simulink model "satellite_GVE_per_model_withMPC_sim"  (R2021a)
settings: Solver=VariableStepAuto  StartTime=0  StopTime=43200  FixedStep=1  RelTol=1e-3
values from neighbouring files (symbols this model uses):
  a = a_ini    (= 7367700)    [Satellite_MPC2.m]
  a_ini = (960e3+1019e3)/2+R_e    (= 7367700)    [Satellite_MPC2.m]
  Cd = 2.2    [Satellite_MPC2.m]
  e = e_ini    (= 0.0039866)    [Satellite_MPC2.m]
  e_ini = 0.0039866    [Satellite_MPC2.m]
  i = i_ini    [Satellite_MPC2.m]
  i_ini = 82.9236/180*pi()    [Satellite_MPC2.m]
  J2 = 1082.63e-6    (= 0.00108263)    [Satellite_MPC2.m]
  K = 2    [Satellite_MPC2.m]
  m_s = 27    [Satellite_MPC2.m]
  meu = G*m_e    (= 397865500000000)    [Satellite_MPC2.m]
  Ohm = Ohm_ini    [Satellite_MPC2.m]
  Ohm_ini = 272.9481/180*pi()    [Satellite_MPC2.m]
  p_solar = 4.65e-06    [Satellite_MPC2.m]
  R_e = 6378.2e3    (= 6378200)    [Satellite_MPC2.m]
  s = 0.2*0.2    (= 0.04)    [Satellite_MPC2.m]
  theta = theta_ini    (= 0)    [Satellite_MPC2.m]
  w = w_ini    [Satellite_MPC2.m]
  w_ini = 297.2910/180*pi()    [Satellite_MPC2.m]
libraries: mpclib x1
settings Model: OrderedModelArguments=off  Creator=18214  LastModifiedBy=18214

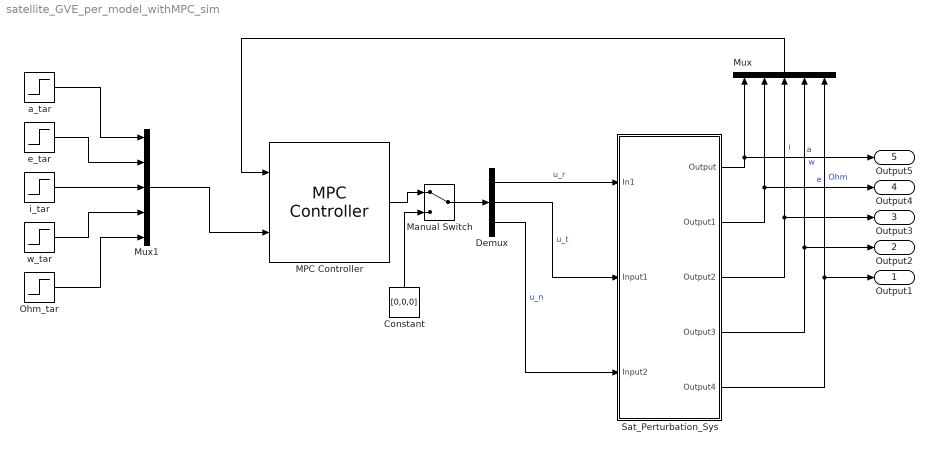
== system satellite_GVE_per_model_withMPC_sim ==
  Constant : Constant  Value=[0,0,0]
  Demux : Demux  Outputs=3
  MPC Controller : mpclib/MPC Controller  SCDEnableBlockLinearizationSpecification=on  mpcobj=mpc_per_exclude  is_multiple=0  enable_value=0  return_u0=off  updateMPCinCallerWorkspace=on  md_inport=off  mv_inport=off  uref_inport=off  return_cost=off  return_mvseq=off  return_qpstatus=off  return_xseq=off  return_state=off  return_ovseq=off  state_inport=off  umin_inport=off  umax_inport=off  ymin_inport=off  ymax_inport=off  cc_inport=off  ywt_inport=off  uwt_inport=off  duwt_inport=off  rhoeps_inport=off  pm_inport=off  MaximumP=10  HorizonChoice=FixedHorizon  n_ts=0.001  n_p=15  n_mv=3  n_md=0  n_ud=0  n_mo=5  n_uo=0  BlockDataType=double  SampleTimeInherited=off  switch_inport=off
  Manual Switch : ManualSwitch
  Mux : Mux  Inputs=5
  Mux1 : Mux  Inputs=5
  Ohm_tar : Step  Time=0  After=Ohm_ini  SampleTime=0
  Sat_Perturbation_Sys : Subsystem
  a_tar : Step  Time=0  After=a_ini  SampleTime=0
  e_tar : Step  Time=0  After=e_ini  SampleTime=0
  i_tar : Step  Time=0  After=i_ini  SampleTime=0
  w_tar : Step  Time=0  After=w_ini  SampleTime=0
  Output1 : Outport
  Output2 : Outport  Port=2
  Output3 : Outport  Port=3
  Output4 : Outport  Port=4
  Output5 : Outport  Port=5
  wires:
  Demux/2 -> Sat_Perturbation_Sys/2(Input1)  "u_t"
  Demux/3 -> Sat_Perturbation_Sys/3(Input2)  "u_n"
  Sat_Perturbation_Sys/1(Output) -> Mux/1, Output5/1  "a"
  Sat_Perturbation_Sys/2(Output1) -> Mux/2, Output4/1  "e"
  Sat_Perturbation_Sys/3(Output2) -> Mux/3, Output3/1  "i"
  Sat_Perturbation_Sys/4(Output3) -> Mux/4, Output2/1  "w"
  Demux/1 -> Sat_Perturbation_Sys/1(In1)  "u_r"
  Sat_Perturbation_Sys/5(Output4) -> Mux/5, Output1/1  "Ohm"
  MPC Controller/1 -> Manual Switch/1
  Mux/1 -> MPC Controller/1
  Mux1/1 -> MPC Controller/2
  a_tar/1 -> Mux1/1
  e_tar/1 -> Mux1/2
  i_tar/1 -> Mux1/3
  w_tar/1 -> Mux1/4
  Ohm_tar/1 -> Mux1/5
  Manual Switch/1 -> Demux/1
  Constant/1 -> Manual Switch/2

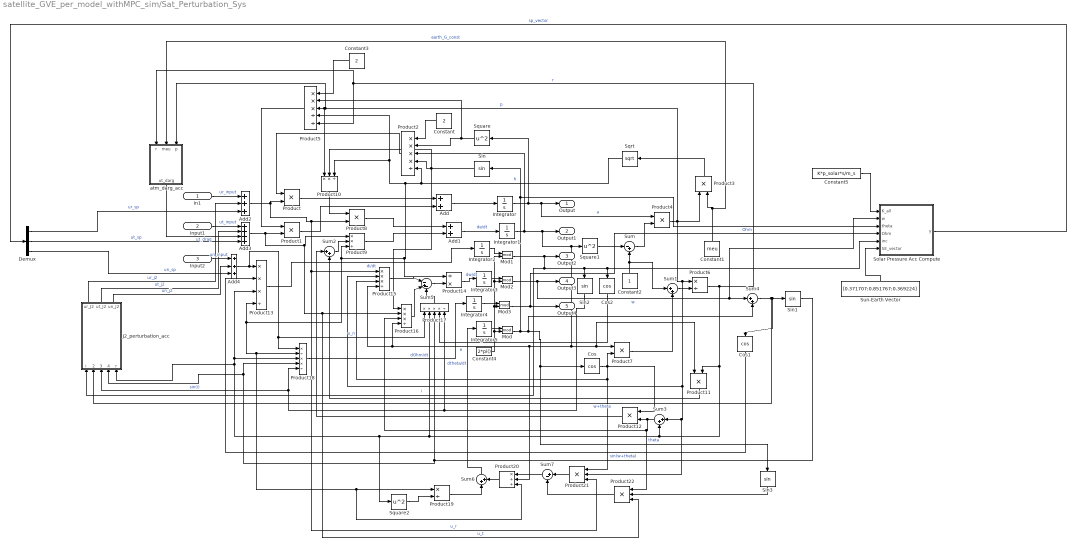
== system satellite_GVE_per_model_withMPC_sim/Sat_Perturbation_Sys ==
  In1 : Inport
  Input1 : Inport  Port=2
  Input2 : Inport  Port=3
  Add : Sum
  Add1 : Sum
  Add2 : Sum  Inputs=+++
  Add3 : Sum  Inputs=++++
  Add4 : Sum  Inputs=+++
  Constant : Constant  Value=2
  Constant1 : Constant  Value=meu
  Constant2 : Constant
  Constant3 : Constant  Value=2
  Constant4 : Constant  Value=2*pi()
  Constant5 : Constant  Value=K*p_solar*s/m_s
  Cos : Trigonometry  Operator=cos
  Cos1 : Trigonometry  Operator=cos
  Cos2 : Trigonometry  Operator=cos
  Demux : Demux  Outputs=3
  Integrator : Integrator  InitialCondition=a  LimitOutput=on  LowerSaturationLimit=R_e
  Integrator1 : Integrator  InitialCondition=e  LimitOutput=on  UpperSaturationLimit=1  LowerSaturationLimit=0
  Integrator2 : Integrator  InitialCondition=i  UpperSaturationLimit=312.5963  LowerSaturationLimit=-312.5963
  Integrator3 : Integrator  InitialCondition=w  UpperSaturationLimit=312.5963  LowerSaturationLimit=-312.5963
  Integrator4 : Integrator  InitialCondition=Ohm  UpperSaturationLimit=312.5963  LowerSaturationLimit=-312.5963
  Integrator5 : Integrator  InitialCondition=theta  UpperSaturationLimit=312.5963  LowerSaturationLimit=-312.5963
  J2_perturbation_acc : Subsystem
  Mod{,1..3} (4 alike) : Math  Operator=mod  SaturateOnIntegerOverflow=on
  Product{,1,3..4,7..8,11..12} (8 alike) : Product
  Product10 : Product  Inputs=**/
  Product13 : Product  Inputs=***/
  Product14 : Product  Inputs=/*
  Product15 : Product  Inputs=***/
  Product16 : Product  Inputs=***/
  Product17 : Product  Inputs=****/
  Product18 : Product  Inputs=*/**/
  Product19 : Product  Inputs=*/
  Product2 : Product  Inputs=****/
  Product20 : Product  Inputs=*//
  Product21 : Product  Inputs=***
  Product22 : Product  Inputs=***
  Product5 : Product  Inputs=***//
  Product6 : Product  Inputs=*/
  Product9 : Product  Inputs=**/
  Sin{,1..3} (4 alike) : Trigonometry
  Solar Pressure Acc Compute : MATLAB Function  TreatAsAtomicUnit=on
  Sqrt : Sqrt  SaturateOnIntegerOverflow=on
  Square : Math  Operator=square  SaturateOnIntegerOverflow=on
  Square1 : Math  Operator=square  SaturateOnIntegerOverflow=on
  Square2 : Math  Operator=square  SaturateOnIntegerOverflow=on
  Sum : Sum  Inputs=|-+
  Sum{1..4,6} (5 alike) : Sum  Inputs=|++
  Sum5 : Sum  Inputs=|-+-
  Sum7 : Sum  Inputs=|+-
  Sun-Earth Vector : Constant  Value=[0.371707;0.851767;0.369224]
  atm_darg_acc : Subsystem
  Output : Outport
  Output1 : Outport  Port=2
  Output2 : Outport  Port=3
  Output3 : Outport  Port=4
  Output4 : Outport  Port=5
  wires:
  Integrator/1 -> Output/1, Product4/1, Square/1  "a"
  Square2/1 -> Product19/2
  Product2/1 -> Product/1
  Mod/1 -> Sin/1, Solar Pressure Acc Compute/3(theta), Sin3/1, Cos/1, Sum4/2  "theta"
  Sin1/1 -> Product18/4, J2_perturbation_acc/4(sin(w+theta)), Product17/3  "sin(w+theta)"
  Product21/1 -> Sum7/1
  Sum5/1 -> Product14/2
  Cos/1 -> Product21/1, Product15/3, Product12/1, Product7/2
  Product4/1 -> Product15/2, Product21/2, Sum3/1, Product6/1, atm_darg_acc/3(p), Product10/1, Product5/3, Product3/1  "p"
  Cos2/1 -> Product17/4
  Sin/1 -> Product16/1, Product10/2, Product2/4
  Sqrt/1 -> Product10/3, Product5/4, Product14/1, Product13/4, Product20/3, Product19/1, Product18/2, Product9/3, Product2/5  "h"
  Product12/1 -> Sum2/1
  Sum/1 -> Product4/2
  Sum3/1 -> Product22/1, Product16/3, Product12/2
  Sum7/1 -> Product20/1
  Product1/1 -> Add/2
  Product22/1 -> Sum7/2
  Add2/1 -> Product/2, Product21/3, Product15/1, Product8/2  "u_r"
  Product7/1 -> Sum1/2
  Product5/1 -> Product1/1
  Sin3/1 -> Product22/2
  Product15/1 -> Sum5/1
  Integrator1/1 -> Product2/3, Output1/1, Square1/1, Product7/1, Product11/1, Product20/2, Product16/4, Product15/4  "e"
  Sum1/1 -> Product6/2
  Cos1/1 -> Product13/2
  Product19/1 -> Sum6/1
  Product8/1 -> Add1/1
  Product6/1 -> atm_darg_acc/1(r), Product5/5, Square2/1, J2_perturbation_acc/5(r), Product13/3, Product18/3, Product17/2, Sum3/2, Product11/2  "r"
  Constant2/1 -> Sum/2, Sum1/1
  Square/1 -> Product5/2, Product2/2
  Product11/1 -> Sum2/2
  Product/1 -> Add/1
  Mod1/1 -> Output2/1, Solar Pressure Acc Compute/5(inc), Cos2/1, Sin2/1, J2_perturbation_acc/1(i)  "i"
  Sin2/1 -> Product18/5, J2_perturbation_acc/3(sin(i)), Product17/5  "sin(i)"
  Product17/1 -> Sum5/3
  Product16/1 -> Sum5/2
  Sum6/1 -> Integrator5/1  "dtheta/dt"
  Product10/1 -> Product8/1
  Product9/1 -> Add1/2
  Sum4/1 -> Sin1/1, Cos1/1, J2_perturbation_acc/2(w+theta)  "w+theta"
  Product20/1 -> Sum6/2
  Mod2/1 -> Solar Pressure Acc Compute/2(w), Sum4/1, Output3/1  "w"
  Add3/1 -> Product22/3, Product16/2, Product9/1, Product1/2  "u_t"
  Constant/1 -> Product2/1
  Sum2/1 -> Product9/2
  Product14/1 -> Integrator3/1  "dw/dt"
  Square1/1 -> Sum/1
  Add4/1 -> Product18/1, Product17/1, Product13/1  "u_n"
  Product13/1 -> Integrator2/1  "di/dt"
  Constant1/1 -> atm_darg_acc/2(meu), Product3/2  "earth_G_const"
  Mod3/1 -> Solar Pressure Acc Compute/4(Ohm), Output4/1  "Ohm"
  Product18/1 -> Integrator4/1  "dOhm/dt"
  Add1/1 -> Integrator1/1  "de/dt"
  Constant3/1 -> Product5/1
  Product3/1 -> Sqrt/1
  Integrator5/1 -> Mod/1
  Constant4/1 -> Mod3/2, Mod2/2, Mod1/2, Mod/2
  In1/1 -> Add2/1  "ur_input"
  Input1/1 -> Add3/1  "ut_input"
  Input2/1 -> Add4/1  "un_input"
  atm_darg_acc/1(ut_darg) -> Add3/3  "ut_drag"
  J2_perturbation_acc/1(ur_J2) -> Add2/2  "ur_j2"
  J2_perturbation_acc/2(ut_J2) -> Add3/2  "ut_j2"
  J2_perturbation_acc/3(un_J2) -> Add4/2  "un_j2"
  Add/1 -> Integrator/1
  Integrator2/1 -> Mod1/1
  Integrator3/1 -> Mod2/1
  Integrator4/1 -> Mod3/1
  Sun-Earth Vector/1 -> Solar Pressure Acc Compute/6(SE_vector)
  Constant5/1 -> Solar Pressure Acc Compute/1(K_all)
  Solar Pressure Acc Compute/1(y) -> Demux/1  "sp_vector"
  Demux/1 -> Add2/3  "ur_sp"
  Demux/2 -> Add3/4  "ut_sp"
  Demux/3 -> Add4/3  "un_sp"

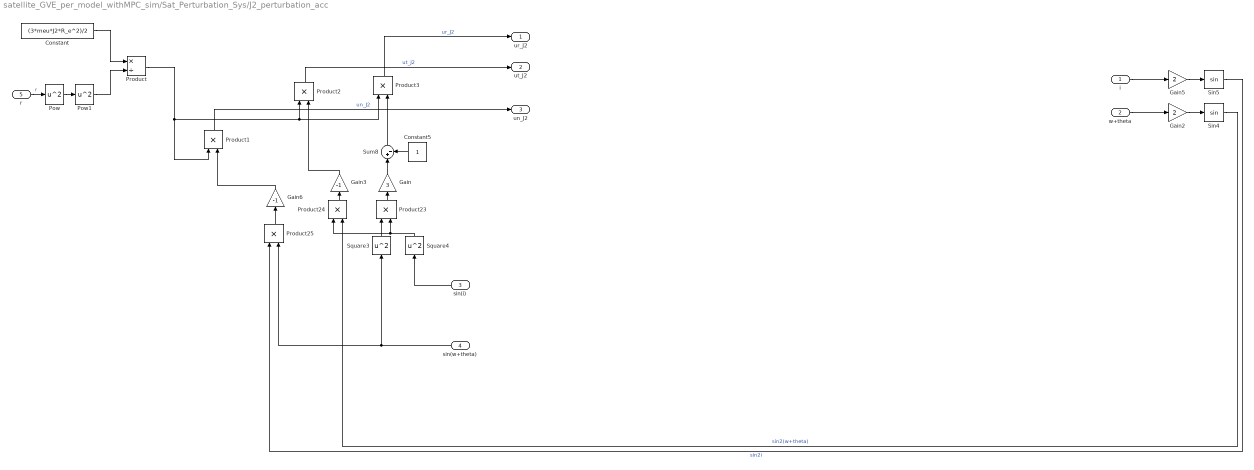
== system satellite_GVE_per_model_withMPC_sim/Sat_Perturbation_Sys/J2_perturbation_acc ==
  i : Inport
  w+theta : Inport  Port=2
  sin(i) : Inport  Port=3
  sin(w+theta) : Inport  Port=4
  r : Inport  Port=5
  Constant : Constant  Value=(3*meu*J2*R_e^2)/2
  Constant5 : Constant
  Gain : Gain  Gain=3
  Gain2 : Gain  Gain=2
  Gain3 : Gain  Gain=-1
  Gain5 : Gain  Gain=2
  Gain6 : Gain  Gain=-1
  Pow : Math  Operator=square  RndMeth=Zero  SaturateOnIntegerOverflow=on
  Pow1 : Math  Operator=square  RndMeth=Zero  SaturateOnIntegerOverflow=on
  Product : Product  Inputs=*/
  Product{1..3,23..25} (6 alike) : Product
  Sin4 : Trigonometry
  Sin5 : Trigonometry
  Square3 : Math  Operator=square  SaturateOnIntegerOverflow=on
  Square4 : Math  Operator=square  SaturateOnIntegerOverflow=on
  Sum8 : Sum  Inputs=|+-
  ur_J2 : Outport
  ut_J2 : Outport  Port=2
  un_J2 : Outport  Port=3
  wires:
  Gain6/1 -> Product1/2
  Square4/1 -> Product23/2, Product24/1
  i/1 -> Gain5/1
  Square3/1 -> Product23/1
  Sin4/1 -> Product24/2  "sin2(w+theta)"
  Sum8/1 -> Product3/2
  Product3/1 -> ur_J2/1  "ur_J2"
  Gain5/1 -> Sin5/1
  Gain3/1 -> Product2/2
  w+theta/1 -> Gain2/1
  Gain/1 -> Sum8/1
  Product23/1 -> Gain/1
  sin(w+theta)/1 -> Product25/2, Square3/1
  Constant5/1 -> Sum8/2
  Sin5/1 -> Product25/1  "sin2i"
  Gain2/1 -> Sin4/1
  Product25/1 -> Gain6/1
  Product24/1 -> Gain3/1
  Product2/1 -> ut_J2/1  "ut_J2"
  sin(i)/1 -> Square4/1
  Product1/1 -> un_J2/1  "un_J2"
  r/1 -> Pow/1  "r"
  Pow1/1 -> Product/2
  Constant/1 -> Product/1
  Product/1 -> Product3/1, Product2/1, Product1/1
  Pow/1 -> Pow1/1

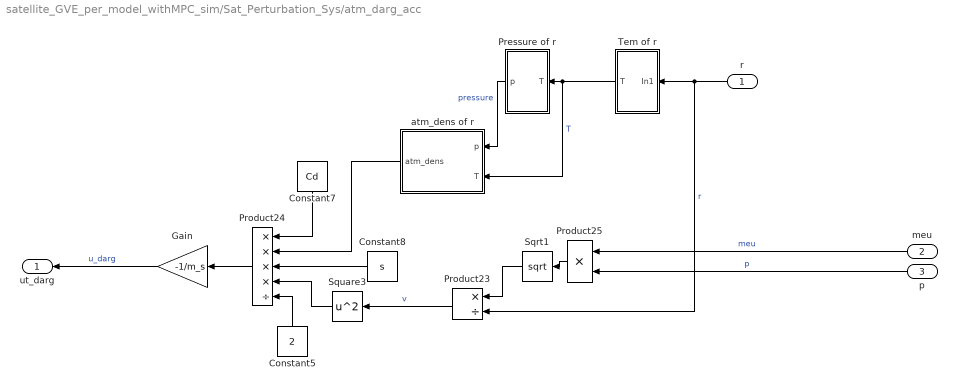
== system satellite_GVE_per_model_withMPC_sim/Sat_Perturbation_Sys/atm_darg_acc ==
  r : Inport
  meu : Inport  Port=2
  p : Inport  Port=3
  Constant5 : Constant  Value=2
  Constant7 : Constant  Value=Cd
  Constant8 : Constant  Value=s
  Gain : Gain  Gain=-1/m_s
  Pressure of r : Subsystem
  Product23 : Product  Inputs=*/
  Product24 : Product  Inputs=****/
  Product25 : Product
  Sqrt1 : Sqrt  SaturateOnIntegerOverflow=on
  Square3 : Math  Operator=square  SaturateOnIntegerOverflow=on
  Tem of r : Subsystem
  atm_dens of r : Subsystem
  ut_darg : Outport
  wires:
  Tem of r/1(T) -> atm_dens of r/2(T), Pressure of r/1(T)  "T"
  Product24/1 -> Gain/1
  r/1 -> Product23/2, Tem of r/1(In1)  "r"
  Product25/1 -> Sqrt1/1
  Square3/1 -> Product24/4
  meu/1 -> Product25/1  "meu"
  Product23/1 -> Square3/1  "v"
  Constant7/1 -> Product24/1
  Sqrt1/1 -> Product23/1
  Pressure of r/1(p) -> atm_dens of r/1(p)  "pressure"
  Constant5/1 -> Product24/5
  atm_dens of r/1(atm_dens) -> Product24/2
  Constant8/1 -> Product24/3
  Gain/1 -> ut_darg/1  "u_darg"
  p/1 -> Product25/2  "p"

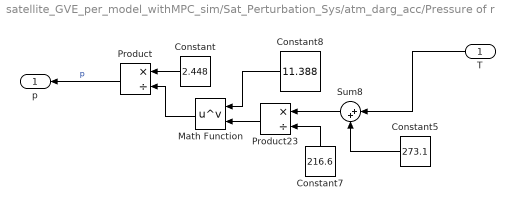
== system satellite_GVE_per_model_withMPC_sim/Sat_Perturbation_Sys/atm_darg_acc/Pressure of r ==
  T : Inport
  Constant : Constant  Value=2.448
  Constant5 : Constant  Value=273.1
  Constant7 : Constant  Value=216.6
  Constant8 : Constant  Value=11.388
  Math Function : Math  Operator=pow  SaturateOnIntegerOverflow=on
  Product : Product  Inputs=*/
  Product23 : Product  Inputs=*/
  Sum8 : Sum  Inputs=|++
  p : Outport
  wires:
  Constant5/1 -> Sum8/2
  Product/1 -> p/1  "p"
  T/1 -> Sum8/1
  Constant8/1 -> Math Function/1
  Sum8/1 -> Product23/1
  Constant7/1 -> Product23/2
  Product23/1 -> Math Function/2
  Math Function/1 -> Product/2
  Constant/1 -> Product/1

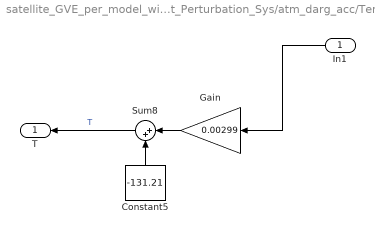
== system satellite_GVE_per_model_withMPC_sim/Sat_Perturbation_Sys/atm_darg_acc/Tem of r ==
  In1 : Inport
  Constant5 : Constant  Value=-131.21
  Gain : Gain  Gain=0.00299
  Sum8 : Sum  Inputs=|++
  T : Outport
  wires:
  Sum8/1 -> T/1  "T"
  Gain/1 -> Sum8/1
  Constant5/1 -> Sum8/2
  In1/1 -> Gain/1

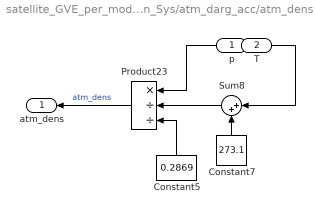
== system satellite_GVE_per_model_withMPC_sim/Sat_Perturbation_Sys/atm_darg_acc/atm_dens of r ==
  p : Inport
  T : Inport  Port=2
  Constant5 : Constant  Value=0.2869
  Constant7 : Constant  Value=273.1
  Product23 : Product  Inputs=*//
  Sum8 : Sum  Inputs=|++
  atm_dens : Outport
  wires:
  T/1 -> Sum8/1
  Constant5/1 -> Product23/3
  Sum8/1 -> Product23/2
  Constant7/1 -> Sum8/2
  Product23/1 -> atm_dens/1  "atm_dens"
  p/1 -> Product23/1

== matlab function satellite_GVE_per_model_withMPC_sim/Sat_Perturbation_Sys/Solar Pressure Acc Compute ==
  data: K_all input; w input; y output; theta input; Ohm input; inc input; SE_vector input
function y = fcn(K_all,w,theta,Ohm,inc,SE_vector)
if((theta>168*pi()/180)&&(theta<278*pi()/180))
    C_oI = zeros(3,3);
    C_rtno = zeros(3,3);
else
    u = w+theta;
    C_oI = [-sin(u)*cos(Ohm)-cos(u)*cos(inc)*sin(Ohm) -sin(u)*sin(Ohm)+cos(u)*cos(inc)*cos(Ohm) cos(u)*sin(inc);
            -sin(inc)*sin(Ohm)                        sin(inc)*cos(Ohm)                         -cos(inc);
            -cos(u)*cos(Ohm)+sin(u)*cos(inc)*sin(Ohm) -cos(u)*sin(Ohm)-sin(u)*cos(inc)*cos(Ohm) -sin(u)*sin(inc)];
    C_rtno = [0 0 -1;1 0 0;0 -1 0];
end
y = K_all*C_rtno*C_oI*SE_vector;
